simulink model "plane"  (R2018b)
settings: Solver=FixedStepAuto  StartTime=0.0  StopTime=inf  FixedStep=0.01  RelTol=1e-3
values from neighbouring files (symbols this model uses):
  A0 = 4.715359540393763e+03    (= 4715.35954039)    [init.m]    (also in test.m = 4713.6877)
  epsilon = deg2rad(90)    [init.m]    (also in test.m = deg2rad(0))
  g = 9.8    [init.m]
  init_plane = [0 3000 0 200 0 deg2rad(-45)]    [init.m]
  init_target = [20000 0 20000]    [init.m]
  omega = deg2rad(3)    [init.m]
  T = 25.46    [init.m]    (also in test.m = 25.45)
  v_wind = 10    [init.m]
settings Model: Creator=ysq  LastModifiedBy=ysq

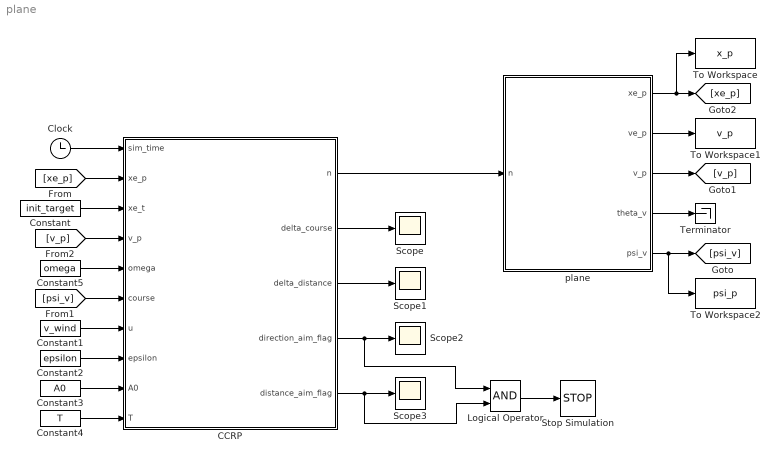
== system plane ==
  CCRP : MATLAB Function  TreatAsAtomicUnit=on
  Clock : Clock
  Constant : Constant  Value=init_target
  Constant1 : Constant  Value=v_wind
  Constant2 : Constant  Value=epsilon
  Constant3 : Constant  Value=A0
  Constant4 : Constant  Value=T
  Constant5 : Constant  Value=omega
  Logical Operator : Logic  AllPortsSameDT=off  OutDataTypeStr=boolean
  Scope{,1..3} (4 alike) : Scope
  Stop Simulation : Stop
  Terminator : Terminator
  To Workspace : ToWorkspace  VariableName=x_p  SampleTime=-1
  To Workspace1 : ToWorkspace  VariableName=v_p  SampleTime=-1
  To Workspace2 : ToWorkspace  VariableName=psi_p  SampleTime=-1
  plane : Subsystem
  wires:
  CCRP/1(n) -> plane/1(n)
  plane/1(xe_p) -> [xe_p], To Workspace/1
  Clock/1 -> CCRP/1(sim_time)
  plane/3(v_p) -> [v_p]
  plane/2(ve_p) -> To Workspace1/1
  [xe_p] -> CCRP/2(xe_p)
  Constant/1 -> CCRP/3(xe_t)
  [psi_v] -> CCRP/6(course)
  plane/4(theta_v) -> Terminator/1
  plane/5(psi_v) -> To Workspace2/1, [psi_v]
  [v_p] -> CCRP/4(v_p)
  Constant1/1 -> CCRP/7(u)
  Constant2/1 -> CCRP/8(epsilon)
  Constant3/1 -> CCRP/9(A0)
  Constant4/1 -> CCRP/10(T)
  Constant5/1 -> CCRP/5(omega)
  CCRP/2(delta_course) -> Scope/1
  CCRP/3(delta_distance) -> Scope1/1
  CCRP/5(distance_aim_flag) -> Logical Operator/2, Scope3/1
  CCRP/4(direction_aim_flag) -> Logical Operator/1, Scope2/1
  Logical Operator/1 -> Stop Simulation/1

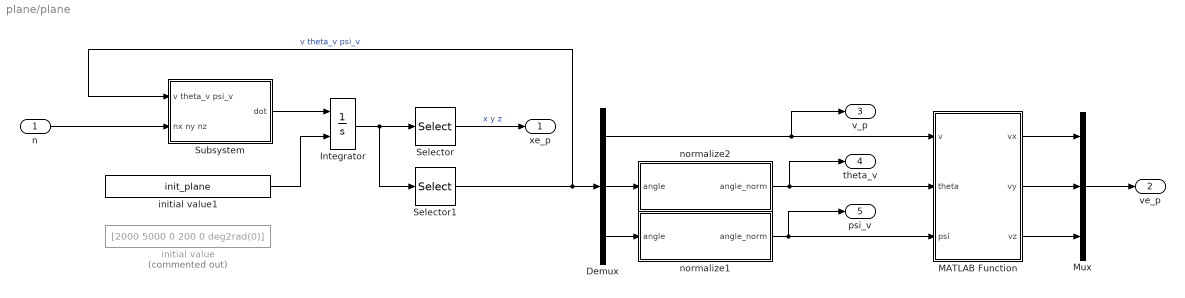
== system plane/plane ==
  n : Inport
  Demux : Demux  Outputs=3
  Integrator : Integrator  InitialConditionSource=external
  MATLAB Function : MATLAB Function  TreatAsAtomicUnit=on
  Mux : Mux  Inputs=3
  Selector : Selector  InputPortWidth=6  IndexOptions=Index vector (dialog)  Indices=[1 2 3]  OutputSizes=1
  Selector1 : Selector  InputPortWidth=6  IndexOptions=Index vector (dialog)  Indices=[4 5 6]  OutputSizes=1
  Subsystem : Subsystem
  initial value : Constant  Commented=on  Value=[2000 5000 0 200 0 deg2rad(0)]
  initial value1 : Constant  Value=init_plane
  normalize1 : MATLAB Function  TreatAsAtomicUnit=on
  normalize2 : MATLAB Function  TreatAsAtomicUnit=on
  xe_p : Outport
  ve_p : Outport  Port=2  PortDimensions=3
  v_p : Outport  Port=3
  theta_v : Outport  Port=4
  psi_v : Outport  Port=5
  wires:
  Selector/1 -> xe_p/1  "x y z"
  n/1 -> Subsystem/2(nx ny nz)
  Subsystem/1(dot) -> Integrator/1
  Integrator/1 -> Selector1/1, Selector/1
  Selector1/1 -> Subsystem/1(v theta_v psi_v), Demux/1  "v theta_v psi_v"
  Demux/1 -> v_p/1, MATLAB Function/1(v)
  Demux/2 -> normalize2/1(angle)
  Demux/3 -> normalize1/1(angle)
  initial value1/1 -> Integrator/2
  normalize1/1(angle_norm) -> psi_v/1, MATLAB Function/3(psi)
  normalize2/1(angle_norm) -> theta_v/1, MATLAB Function/2(theta)
  MATLAB Function/1(vx) -> Mux/1
  MATLAB Function/3(vz) -> Mux/3
  MATLAB Function/2(vy) -> Mux/2
  Mux/1 -> ve_p/1

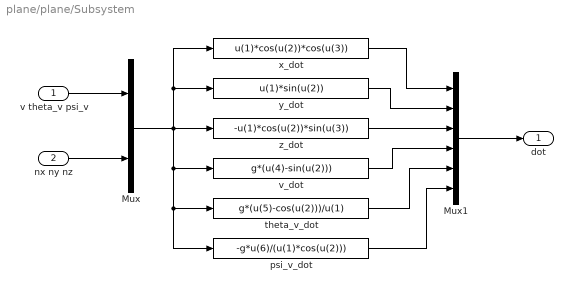
== system plane/plane/Subsystem ==
  v theta_v psi_v : Inport
  nx ny nz : Inport  Port=2
  Mux : Mux  Inputs=2
  Mux1 : Mux  Inputs=6
  psi_v_dot : Fcn  Expr=-g*u(6)/(u(1)*cos(u(2)))
  theta_v_dot : Fcn  Expr=g*(u(5)-cos(u(2)))/u(1)
  v_dot : Fcn  Expr=g*(u(4)-sin(u(2)))
  x_dot : Fcn  Expr=u(1)*cos(u(2))*cos(u(3))
  y_dot : Fcn  Expr=u(1)*sin(u(2))
  z_dot : Fcn  Expr=-u(1)*cos(u(2))*sin(u(3))
  dot : Outport
  wires:
  theta_v_dot/1 -> Mux1/5
  psi_v_dot/1 -> Mux1/6
  Mux1/1 -> dot/1
  y_dot/1 -> Mux1/2
  Mux/1 -> psi_v_dot/1, theta_v_dot/1, v_dot/1, y_dot/1, x_dot/1, z_dot/1
  x_dot/1 -> Mux1/1
  v_dot/1 -> Mux1/4
  z_dot/1 -> Mux1/3
  nx ny nz/1 -> Mux/2
  v theta_v psi_v/1 -> Mux/1

== matlab function plane/CCRP ==
  settings: updateMethod=DISCRETE
  data: sim_time input; n output; xe_p input; xe_t input; v_p input; omega input; course input; u input; epsilon input; A0 input; T input; delta_course output; delta_distance output; direction_aim_flag output; distance_aim_flag output
function [n,delta_course,delta_distance,direction_aim_flag,distance_aim_flag] = ccrp(sim_time,xe_p,xe_t,v_p,omega,course,u,epsilon,A0,T)
persistent direction_aim_complete;
persistent distance_aim_complete;
if isempty(direction_aim_complete)
    direction_aim_complete=0;
end
if isempty(distance_aim_complete)
    distance_aim_complete=0;
end
n=[0,1,0];
delta_course=-1;
delta_distance=-1;

if sim_time>=50 && (~direction_aim_complete || ~distance_aim_complete)
    %direction aim
    dx_nse=xe_t(1)-xe_p(1);
    dz_nse=xe_t(3)-xe_p(3);
    alpha=atan(u*sin(epsilon)/(v_p+u*cos(epsilon)));
    [dx_gs,~]=nse2gs(dx_nse,dz_nse,course,alpha);
    [ax_gs,az_gs] = course2gs(A0,T,u,epsilon,alpha,course);
    if ~direction_aim_complete
        delta_course = direction_aim(course,alpha,dx_nse,dz_nse,dx_gs,az_gs)*57.3;
        if abs(delta_course)>0.01
            if delta_course>0
                n=[0,1,-omega*v_p/9.8];
            else
                n=[0,1,omega*v_p/9.8];
            end
        else
            direction_aim_complete=1;
        end
    end
    %distance aim
    if direction_aim_complete && ~distance_aim_complete
        delta_distance = distance_aim(ax_gs,az_gs,dx_gs);
        if abs(delta_distance)<1
            distance_aim_complete=1;
        end
    end
end
direction_aim_flag=direction_aim_complete;
distance_aim_flag=distance_aim_complete;
end

== matlab function plane/MATLAB Function ==
  data: v input; vx output; theta input; psi input; vy output; vz output
function [vx,vy,vz] = v2ve(v, theta, psi)
vx = v * cos(theta) * cos(psi);      
vy = v * sin(theta);      
vz = -v * cos(theta) * sin(psi);
end

== matlab function plane/normalize1 ==
  data: angle input; angle_norm output
function angle_norm = normalize(angle)
    angle = rad2deg(angle);
    if angle > 180
        angle_norm = angle - floor((angle-(-180))/360)*360;
    elseif angle <= -180
        angle_norm = angle + floor((180-angle)/360)*360;
    else
        angle_norm = angle;
    end
    angle_norm = deg2rad(angle_norm);
end

== matlab function plane/normalize2 ==
  data: angle input; angle_norm output
function angle_norm = normalize(angle)
    angle = rad2deg(angle);
    if angle > 180
        angle_norm = angle - floor((angle-(-180))/360)*360;
    elseif angle <= -180
        angle_norm = angle + floor((180-angle)/360)*360;
    else
        angle_norm = angle;
    end
    angle_norm = deg2rad(angle_norm);
end
